simulink library "simulink"  (R2014a)
settings: Solver=ode45  SolverMode=SingleTasking  StartTime=0.0  StopTime=10.0  RelTol=1e-3
PostLoadFcn:
  | setsysloc_simulink(bdroot)
undefined symbols (not defined in the file or in its folder): DiscIntNeverNeededParam, getdatatypespecs, NumBits1, NumBits2, sfunxy, sigbuilder_block, slcm, SlDemoSign, Slope1, Slope2
libraries: simulink x40, sl_helperblocks x2, eml_lib x1
(part 3 of 5)

== system simulink/Model-Wide Utilities ==
  note: Linearization of Running Models
  note: Documentation
  note: Modeling Guides
  Block Support Table : Subsystem  mask(Block Support Table){}
      mask help: Simulink:masks:BlockSupportTable_MD
      settings: OpenFcn=showblockdatatypetable
      mask Display: disp('Block Support\nTable');
  DocBlock : Subsystem  mask(DocBlock){ECoderFlag=, DocumentType=Text}
      mask prompts: ECoderFlag "Simulink:masks:DocBlockEmbeddedCoderFlagLabel_MP"; DocumentType "Simulink:masks:DocBlockDocTypeLabel_MP"
      mask help: Simulink:masks:DocBlock_MD
      settings: DeleteFcn=docblock('close_document',gcb);  PreSaveFcn=docblock('save_document',gcb);  OpenFcn=docblock('edit_document',gcb);
      mask TypeOptions DocumentType: Simulink:masks:Text | Simulink:masks:RTF | Simulink:masks:HTML
      mask Display:
      | plot([.8 0 0 1 1 .8 .8 1],[1 1 0 0 .8 1 .8 .8]);
      | text(.5,.6,'DOC','horizontalalignment','center');
      | text(.95,.05,get_param(gcb,'DocumentType'),'verticalalignment','bottom','horizontalalignment','right');
  Model Info : Subsystem  LoadFcn=slcm LoadBlock;  InitFcn=slcm('UpdateAllCMBlocksInThisModelInit')  mask(CMBlock){InitialSaveTempField=, InitialBlockCM=None, BlockCM=none, Frame=on, SaveTempField=, DisplayStringWithTags=Model Info, MaskDisplayString=Model Info, HorizontalTextAlignment=Center, LeftAlignmentValue=0.5, SourceBlockDiagram=simulink, TagMaxNumber=20, CMTag1=, CMTag2=, CMTag3=, CMTag4=, CMTag5=, CMTag6=, CMTag7=, CMTag8=, CMTag9=, CMTag10=, CMTag11=, CMTag12=, CMTag13=, CMTag14=, CMTag15=, CMTag16=, CMTag17=, CMTag18=, CMTag19=, CMTag20=}
      mask prompts: InitialSaveTempField "Simulink:masks:InitialSaveTempField_MP"; InitialBlockCM "Simulink:masks:InitialBlockCM_MP"; BlockCM "Simulink:masks:BlockCM_MP"; Frame "Simulink:masks:Frame_MP"; SaveTempField "Simulink:masks:SaveTempField_MP"; DisplayStringWithTags "Simulink:masks:DisplayStringWithTags_MP"; MaskDisplayString "Simulink:masks:MaskDisplayString_MP"; HorizontalTextAlignment "Simulink:masks:HorizontalTextAlignment_MP"; LeftAlignmentValue "Simulink:masks:LeftAlignmentValue_MP"; SourceBlockDiagram "Simulink:masks:SourceBlockDiagram_MP"; TagMaxNumber "Simulink:masks:TagMaxNumber_MP"; CMTag1 "Simulink:masks:CMTag1_MP"; CMTag2 "Simulink:masks:CMTag2_MP"; CMTag3 "Simulink:masks:CMTag3_MP"; CMTag4 "Simulink:masks:CMTag4_MP"; CMTag5 "Simulink:masks:CMTag5_MP"; CMTag6 "Simulink:masks:CMTag6_MP"; CMTag7 "Simulink:masks:CMTag7_MP"; CMTag8 "Simulink:masks:CMTag8_MP"; CMTag9 "Simulink:masks:CMTag9_MP"; CMTag10 "Simulink:masks:CMTag10_MP"; CMTag11 "Simulink:masks:CMTag11_MP"; CMTag12 "Simulink:masks:CMTag12_MP"; CMTag13 "Simulink:masks:CMTag13_MP"; CMTag14 "Simulink:masks:CMTag14_MP"; CMTag15 "Simulink:masks:CMTag15_MP"; CMTag16 "Simulink:masks:CMTag16_MP"; CMTag17 "Simulink:masks:CMTag17_MP"; CMTag18 "Simulink:masks:CMTag18_MP"; CMTag19 "Simulink:masks:CMTag19_MP"; CMTag20 "Simulink:masks:CMTag20_MP"
      mask help: Simulink:masks:CMBlock_MD
      settings: CopyFcn=slcm CopyBlock;  DeleteFcn=slcm Cancel;  PostSaveFcn=slcm('UpdateAllCMBlocksInThisModel')  NameChangeFcn=slcm Rename;  OpenFcn=slcm
      mask Display: text(slResolve(LeftAlignmentValue, gcbh), 0.5, MaskDisplayString, 'HorizontalAlignment', HorizontalTextAlignment)
  Timed-Based Linearization : Subsystem  mask(Timed Linearization){LinearizationTime=1, SampleTime=0}
      mask prompts: LinearizationTime "Simulink:masks:LinearizationTime_MP"; SampleTime "Simulink:masks:SampleTimeofLinearizedModel_MP"
      mask help: Simulink:masks:TimedLinearization_MD
      mask init:
      | name_  = linsetup;
      mask Help: This block calls LINMOD or DLINMOD to create a linear model for the system when the simulation clock reaches the time specified by the LinearizationTime parameter.  No trimming is performed.  The linear model is stored in the base workspace as a structure, along with information about the operating point at which the snapshot was taken.  Multiple snapshots are appended to form an array of structures.
      mask Display: disp(['T=' mat2str(double(LinearizationTime))])
  Trigger-Based Linearization : Subsystem  TreatAsAtomicUnit=on  mask(Triggered Linearization){TriggerType=rising, SampleTime=0}
      mask prompts: TriggerType "Simulink:masks:TriggerType_MP"; SampleTime "Simulink:masks:SampleTimeofLinearizedModel_MP"
      mask help: Simulink:masks:TriggeredLinearization_MD
      mask init:
      | name_ = linsetup;
      | set_param([ gcb '/Trigger'],'TriggerType',TriggerType);
      mask Help: When triggered, this block calls LINMOD or DLINMOD to create a linear model for the system at the current operating point.  No trimming is performed.   The linear model is stored in the base workspace as a structure, along with information about the operating point at which the snapshot was taken.  Multiple snapshots are appended to form an array of structures.
      mask TypeOptions TriggerType: Simulink:masks:rising | Simulink:masks:falling | Simulink:masks:either | Simulink:masks:functionCall

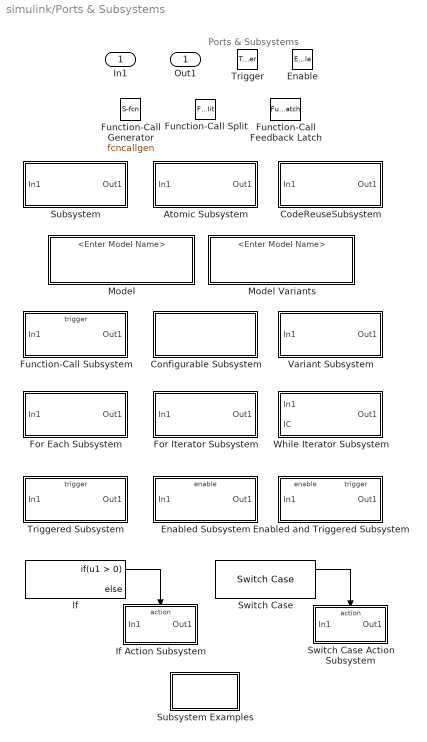
== system simulink/Ports & Subsystems ==
  note: Ports & Subsystems
  In1 : Inport
  Enable : EnablePort
  Trigger : TriggerPort  PortDimensions=1
  Atomic Subsystem : Subsystem  TreatAsAtomicUnit=on  mask(Atomic Subsystem){}
      mask help: Simulink:masks:IOPortSubsystem_MD
      settings: CopyFcn=set_param(gcbh,'LinkStatus','none'); set_param(gcbh,'Mask','off'); set_param(gcbh,'MaskType',''); set_param(gcbh,'MaskDescription',''); set_param(gcbh,'OpenFcn',''); set_param(gcbh,'CopyFcn','')  OpenFcn=open_system(gcbh,'force')
  CodeReuseSubsystem : Subsystem  TreatAsAtomicUnit=on  mask(Code Reuse Subsystem){}
      mask help: Simulink:masks:IOPortSubsystem_MD
      settings: CopyFcn=set_param(gcbh,'LinkStatus','none'); set_param(gcbh,'Mask','off'); set_param(gcbh,'MaskType',''); set_param(gcbh,'MaskDescription',''); set_param(gcbh,'OpenFcn',''); set_param(gcbh,'CopyFcn','')  OpenFcn=open_system(gcb,'force')  RTWFcnNameOpts=Use subsystem name  RTWFileNameOpts=Use function name
  Configurable Subsystem : Subsystem
      settings: TemplateBlock=master
  Enabled Subsystem : Subsystem  TreatAsAtomicUnit=on  mask(Enabled Subsystem){}
      mask help: Simulink:masks:EnabledSubsystem_MD
      settings: CopyFcn=set_param(gcbh,'LinkStatus','none'); set_param(gcbh,'Mask','off'); set_param(gcbh,'MaskType',''); set_param(gcbh,'MaskDescription',''); set_param(gcbh,'OpenFcn',''); set_param(gcbh,'CopyFcn','')  OpenFcn=open_system(gcbh,'force')
  Enabled and Triggered Subsystem : Subsystem  TreatAsAtomicUnit=on  mask(Enabled And Triggered Subsystem){}
      mask help: Simulink:masks:EnabledAndTriggeredSubsystem_MD
      settings: CopyFcn=set_param(gcbh,'LinkStatus','none'); set_param(gcbh,'Mask','off'); set_param(gcbh,'MaskType',''); set_param(gcbh,'MaskDescription',''); set_param(gcbh,'OpenFcn',''); set_param(gcbh,'CopyFcn','')  OpenFcn=open_system(gcbh,'force')
  For Each Subsystem : Subsystem  TreatAsAtomicUnit=on  mask(For Each Subsystem){}
      mask help: Simulink:masks:ForEachSubsystem_MD
      settings: CopyFcn=set_param(gcbh,'LinkStatus','none'); set_param(gcbh,'Mask','off'); set_param(gcbh,'MaskType',''); set_param(gcbh,'MaskDescription',''); set_param(gcbh,'OpenFcn',''); set_param(gcbh,'CopyFcn','')  OpenFcn=open_system(gcbh,'force')
  For Iterator Subsystem : Subsystem  TreatAsAtomicUnit=on  mask(For Iterator Subsystem){}
      mask help: Simulink:masks:ForIteratorSubsystem_MD
      settings: CopyFcn=set_param(gcbh,'LinkStatus','none'); set_param(gcbh,'Mask','off'); set_param(gcbh,'MaskType',''); set_param(gcbh,'MaskDescription',''); set_param(gcbh,'OpenFcn',''); set_param(gcbh,'CopyFcn','')  OpenFcn=open_system(gcbh,'force')
  Function-Call Feedback Latch : FunctionCallFeedbackLatch
  Function-Call Generator : S-Function  FunctionName=fcncallgen  Parameters=sample_time,numberOfIterations  EnableBusSupport=off  mask(Function-Call Generator){sample_time=1, numberOfIterations=1}
      mask prompts: sample_time "Simulink:masks:SampleTime_MP"; numberOfIterations "Simulink:masks:NumberOfIterations_MP"
      mask help: Simulink:masks:FunctionCallGenerator_MD
      mask init:
      | if ~isempty(numberOfIterations) & length(numberOfIterations) == 1 & (numberOfIterations > 1),
      | str=sprintf('iterate I = 1:%d',numberOfIterations);
      | else, str = 'f()';
      | end;
      mask Help: This block executes a function-call subsystem at the rate specified by the sample time and a specified number of times.
      mask Display: disp(str)
  Function-Call Split : FunctionCallSplit
      settings: CopyFcn=set_param(gcbh,'ShowName','off','CopyFcn','')
  Function-Call Subsystem : Subsystem  TreatAsAtomicUnit=on  mask(Function-Call Subsystem){}
      mask help: Simulink:masks:FunctionCallSubsystem_MD
      settings: CopyFcn=set_param(gcbh,'LinkStatus','none'); set_param(gcbh,'Mask','off'); set_param(gcbh,'MaskType',''); set_param(gcbh,'MaskDescription',''); set_param(gcbh,'OpenFcn',''); set_param(gcbh,'CopyFcn','')  OpenFcn=open_system(gcbh,'force')
  If : If
  If Action Subsystem : Subsystem  TreatAsAtomicUnit=on  mask(If Action Subsystem){}
      mask help: Simulink:masks:ActionSubsystem_MD
      settings: CopyFcn=set_param(gcbh,'LinkStatus','none'); set_param(gcbh,'Mask','off'); set_param(gcbh,'MaskType',''); set_param(gcbh,'MaskDescription',''); set_param(gcbh,'OpenFcn',''); set_param(gcbh,'CopyFcn','')  OpenFcn=open_system(gcbh,'force')
  Model : ModelReference  ModelNameDialog=<Enter Model Name>  SimulationMode=Normal  DefaultDataLogging=on
  Model Variants : ModelReference  ModelNameDialog=<Enter Model Name>  SimulationMode=Normal  Variant=on  DefaultDataLogging=on
      settings: AttributesFormatString=%<ActiveVariant>
  Subsystem : Subsystem  mask(Virtual Subsystem){}
      mask help: Simulink:masks:IOPortSubsystem_MD
      settings: CopyFcn=set_param(gcbh,'LinkStatus','none'); set_param(gcbh,'Mask','off'); set_param(gcbh,'MaskType',''); set_param(gcbh,'MaskDescription',''); set_param(gcbh,'OpenFcn',''); set_param(gcbh,'CopyFcn','')  OpenFcn=open_system(gcbh,'force')
  Subsystem Examples : Subsystem  mask(Subsystem Examples){}
      mask help: Simulink:masks:SubsystemExamples_MD
      settings: OpenFcn=open_system('sl_subsys_semantics','force')
      mask Display: disp('Subsystem\nExamples')
  Switch Case : SwitchCase
  Switch Case Action Subsystem : Subsystem  TreatAsAtomicUnit=on  mask(Switch Case Action Subsystem){}
      mask help: Simulink:masks:ActionSubsystem_MD
      settings: CopyFcn=set_param(gcbh,'LinkStatus','none'); set_param(gcbh,'Mask','off'); set_param(gcbh,'MaskType',''); set_param(gcbh,'MaskDescription',''); set_param(gcbh,'OpenFcn',''); set_param(gcbh,'CopyFcn','')  OpenFcn=open_system(gcbh,'force')
  Triggered Subsystem : Subsystem  TreatAsAtomicUnit=on  mask(Triggered Subsystem){}
      mask help: Simulink:masks:TriggeredSubsystem_MD
      settings: CopyFcn=set_param(gcbh,'LinkStatus','none'); set_param(gcbh,'Mask','off'); set_param(gcbh,'MaskType',''); set_param(gcbh,'MaskDescription',''); set_param(gcbh,'OpenFcn',''); set_param(gcbh,'CopyFcn','')  OpenFcn=open_system(gcbh,'force')
  Variant Subsystem : Subsystem  Variant=on  mask(Variant Subsystem){}
      mask help: Simulink:masks:VariantSubsystem_MD
      settings: CopyFcn=set_param(gcbh,'LinkStatus','none'); set_param(gcbh,'Mask','off'); set_param(gcbh,'MaskType',''); set_param(gcbh,'MaskDescription',''); set_param(gcbh,'OpenFcn',''); set_param(gcbh,'CopyFcn','')
  While Iterator Subsystem : Subsystem  TreatAsAtomicUnit=on  mask(While Iterator Subsystem){}
      mask help: Simulink:masks:WhileIteratorSubsystem_MD
      settings: CopyFcn=set_param(gcbh,'LinkStatus','none'); set_param(gcbh,'Mask','off'); set_param(gcbh,'MaskType',''); set_param(gcbh,'MaskDescription',''); set_param(gcbh,'OpenFcn',''); set_param(gcbh,'CopyFcn','')  OpenFcn=open_system(gcbh,'force')
  Out1 : Outport
  wires:
  If/1 -> If Action Subsystem/Action
  Switch Case/1 -> Switch Case Action Subsystem/Action

== system simulink/Signal Attributes ==
  note: Signal Attribute Manipulation
  note: Signal Attribute Detection
  Bus to Vector : BusToVector
  Data Type Conversion Inherited : Subsystem  mask(Conversion Inherited){ConvertRealWorld=Real World Value, RndMeth=Floor, DoSatur=off}
      mask prompts: ConvertRealWorld "Simulink:masks:InputAndOutputToHaveEqual_MP"; RndMeth "Simulink:masks:IntegerRoundingMode_MP"; DoSatur "Simulink:masks:SaturateToMaxOrMinWhenOverflowsOccur_MP"
      mask help: Simulink:masks:ConversionInherited_MD
      mask init:
      | rndMethCell = {'Ceiling','Convergent','Floor','Nearest','Round','Simplest','Zero'};
      | onOffCell = {'off','on'};
      | RWVvsSICell = { 'Real World Value','Stored Integer'};
      | set_param([gcb,'/Conversion'],'RndMeth',rndMethCell{RndMeth},...
      |                                 'DoSatur',onOffCell{DoSatur+1},...
      |                                 'ConvertRealWorld',RWVvsSICell{ConvertRealWorld});
      mask TypeOptions ConvertRealWorld: Simulink:masks:RealWorldValue | Simulink:masks:StoredInteger
      mask TypeOptions RndMeth: Simulink:masks:Ceiling | Simulink:masks:Convergent | Simulink:masks:Floor | Simulink:masks:Nearest | Simulink:masks:Round | Simulink:masks:Simplest | Simulink:masks:Zero
      mask Display:
      | port_label('Input',2,'u');
      | port_label('Output',1,'y');
      | disp('Convert')
  Data Type Duplicate : DataTypeDuplicate
  Data Type Propagation : S-Function  FunctionName=sfix_dtprop  Parameters=14,PropDataTypeMode,(getdatatypespecs(PropDataType,PropScaling,DblOver,0, 0, PropDataTypeMode, PropScalingMode)),IfRefDouble,IfRefSingle,IsSigned,NumBitsBase,NumBitsMult,NumBitsAdd,(sort(reshape(round(NumBitsAllowFinal), prod(size(NumBitsAllowFinal)),1))),PropScalingMode,ValuesUsedBestPrec,SlopeBase,SlopeMult,SlopeAdd,BiasBase,BiasMult,BiasAdd,DblOver  EnableBusSupport=off  mask(Data Type Propagation){PropDataTypeMode=Inherit via propagation rule, PropDataType=fixdt(1, 16), IfRefDouble=double, IfRefSingle=single, IsSigned=IsSigned1 or IsSigned2, NumBitsBase=max([NumBits1 NumBits2]), NumBitsMult=1, NumBitsAdd=0, NumBitsAllowFinal=1:128, PropScalingMode=Inherit via propagation rule, PropScaling=2^-10, ValuesUsedBestPrec=[5 -7], SlopeBase=min([Slope1 Slope2]), SlopeMult=1, SlopeAdd=0, BiasBase=Bias1, BiasMult=1, BiasAdd=0}
      mask prompts: PropDataTypeMode "Simulink:masks:x1PropagatedDataType_MP"; PropDataType "Simulink:masks:x11PropagatedDataTypeegFixdt116Fixdtsingle_MP"; IfRefDouble "Simulink:masks:x11IfAnyReferenceInputIsDoubleOutputIs_MP"; IfRefSingle "Simulink:masks:x12IfAnyReferenceInputIsSingleOutputIs_MP"; IsSigned "Simulink:masks:x13IsSigned_MP"; NumBitsBase "Simulink:masks:x141NumberofBitsBase_MP"; NumBitsMult "Simulink:masks:x142NumberofBitsMultiplicativeAdjustment_MP"; NumBitsAdd "Simulink:masks:x143NumberofBitsAdditiveAdjustment_MP"; NumBitsAllowFinal "Simulink:masks:x144NumberofBitsAllowableFinalValues_MP"; PropScalingMode "Simulink:masks:x2PropagatedScaling_MP"; PropScaling "Simulink:masks:x21PropagatedScalingSlopeEg29OrSlopeBiasEg1253_MP"; ValuesUsedBestPrec "Simulink:masks:x21ValuesUsedToDetermineBestPrecisionScaling_MP"; SlopeBase "Simulink:masks:x211SlopeBase_MP"; SlopeMult "Simulink:masks:x212SlopeMultiplicativeAdjustment_MP"; SlopeAdd "Simulink:masks:x213SlopeAdditiveAdjustment_MP"; BiasBase "Simulink:masks:x221BiasBase_MP"; BiasMult "Simulink:masks:x222BiasMultiplicativeAdjustment_MP"; BiasAdd "Simulink:masks:x223BiasAdditiveAdjustment_MP"
      mask help: Simulink:masks:DataTypePropagation_MD
      mask init:
      | DblOver = 0;
      mask TypeOptions PropDataTypeMode: Simulink:masks:SpecifyViaDialog | Simulink:masks:InheritViaPropagationRule
      mask Callback PropDataTypeMode: fixptdialog(gcbh)
      mask Callback PropDataType: fixptdialog(gcbh)
      mask TypeOptions IfRefDouble: Simulink:masks:double | Simulink:masks:single
      mask TypeOptions IfRefSingle: Simulink:masks:double | Simulink:masks:single
      mask TypeOptions IsSigned: Simulink:masks:IsSigned1 | Simulink:masks:IsSigned2 | Simulink:masks:IsSigned1OrIsSigned2 | Simulink:masks:TRUE | Simulink:masks:FALSE
      mask TypeOptions NumBitsBase: NumBits1 | NumBits2 | max([NumBits1 NumBits2]) | min([NumBits1 NumBits2]) | NumBits1+NumBits2
      mask TypeOptions PropScalingMode: Simulink:masks:SpecifyViaDialog | Simulink:masks:InheritViaPropagationRule | Simulink:masks:ObtainViaBestPrecision
      mask Callback PropScalingMode: fixptdialog(gcbh)
      mask TypeOptions SlopeBase: Slope1 | Slope2 | max([Slope1 Slope2]) | min([Slope1 Slope2]) | Slope1*Slope2 | Slope1/Slope2 | PosRange1 | PosRange2 | max([PosRange1 PosRange2]) | min([PosRange1 PosRange2]) | PosRange1*PosRange2 | PosRange1/PosRange2
      mask TypeOptions BiasBase: Bias1 | Bias2 | max([Bias1 Bias2]) | min([Bias1 Bias2]) | Bias1*Bias2 | Bias1/Bias2 | Bias1+Bias2 | Bias1-Bias2
      mask Display:
      | port_label('Input',1,'Ref1');
      | port_label('Input',2,'Ref2');
      | port_label('Input',3,'Prop');
  Data Type Propagation Examples : Subsystem  mask(Data Type Propagation Examples){}
      mask help: Simulink:masks:DataTypePropagationExamples_MD
      settings: OpenFcn=open_system('fixpt_dtprop','force')
      mask Display: disp('Data Type\nPropagation\nExamples')
  Data Type Scaling Strip : Subsystem  mask(Scaling Strip){}
      mask help: Simulink:masks:ScalingStrip_MD
      mask Display: fprintf('Scaling\nStrip')
  Data Type Conversion : DataTypeConversion
  IC : InitialCondition
  Probe : Probe  ProbeSignalDimensions=on  ProbeFramedSignal=on
  Rate Transition : RateTransition
  Signal Conversion : SignalConversion
  Signal Specification : SignalSpecification
  Weighted Sample Time : SampleTimeMath  TsampMathOp=Ts Only
  Width : Width

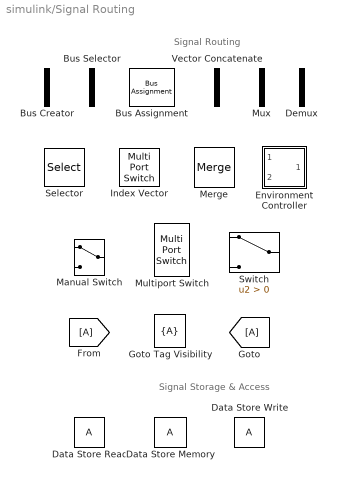
== system simulink/Signal Routing ==
  note: Signal Routing
  note: Signal Storage & Access
  Bus Assignment : BusAssignment
  Bus Creator : BusCreator  Inputs=2
      settings: CopyFcn=set_param(gcbh,'ShowName','off','CopyFcn','')
  Bus Selector : BusSelector  OutputSignals=signal1,signal2
      settings: CopyFcn=set_param(gcbh,'ShowName','off','CopyFcn','')
  Data Store Memory : DataStoreMemory  ReadBeforeWriteMsg=warning  WriteAfterWriteMsg=warning  WriteAfterReadMsg=warning
  Data Store Read : DataStoreRead
  Data Store Write : DataStoreWrite
  Demux : Demux  Outputs=2
      settings: CopyFcn=set_param(gcbh,'ShowName','off','CopyFcn','')
  Environment Controller : Subsystem  mask(Environment Controller){}
      mask help: Simulink:masks:EnvironmentController_MD
      mask init:
      | switch_mode = rtwenvironmentmode(bdroot(gcbh)) || ...
      |     (exist('sldvisactive','file')~=0 && sldvisactive(bdroot(gcbh)));
  Goto Tag Visibility : GotoTagVisibility
  Index Vector : MultiPortSwitch  DataPortOrder=Zero-based contiguous  Inputs=1  zeroidx=on
  Manual Switch : ManualSwitch
  Merge : Merge
  Multiport Switch : MultiPortSwitch
  Mux : Mux  Inputs=2
      settings: CopyFcn=set_param(gcbh,'ShowName','off','CopyFcn','')
  Selector : Selector  InputPortWidth=3  Indices=[1 3]
  Switch : Switch  Criteria=u2 > Threshold
  Vector Concatenate : Concatenate

== system simulink/Sinks ==
  note: Model & Subsystem Outputs
  note: Simulation Control
  note: Data Viewers
  Display : Display
  Floating Scope : Scope
      settings: Floating=on
  Scope : Scope
  Stop Simulation : Stop
  Terminator : Terminator
  To File : ToFile  SaveFormat=Timeseries
  To Workspace : ToWorkspace  VariableName=simout  SaveFormat=Timeseries  SampleTime=-1
  XY Graph : Subsystem  LoadFcn=sfunxy([],[],[],'LoadBlock')  StartFcn=sfunxy([],[],[],'Start')  StopFcn=sfunxy([],[],[],'Stop')  TreatAsAtomicUnit=on  SimViewingDevice=on  mask(XY scope.){xmin=-1, xmax=1, ymin=-1, ymax=1, st=-1}
      mask prompts: xmin "Simulink:masks:xmin_MP"; xmax "Simulink:masks:xmax_MP"; ymin "Simulink:masks:ymin_MP"; ymax "Simulink:masks:ymax_MP"; st "Simulink:masks:SampleTime_MP"
      mask help: Simulink:masks:XYScope_MD
      settings: CopyFcn=sfunxy([],[],[],'CopyBlock')  DeleteFcn=sfunxy([],[],[],'DeleteBlock')  NameChangeFcn=sfunxy([],[],[],'NameChange')
      mask Help: This block can be used to explore limit cycles. Look at the m-file sfunxy.m to see how it works.
      mask Display: plot([.05 .95 .95 .05 .05],[.45 .45 .95 .95 .45], 0.5+cos(0:0.1:2*pi)*0.3,0.7+sin(0:0.1:2*pi)*0.2)
  Out1 : Outport

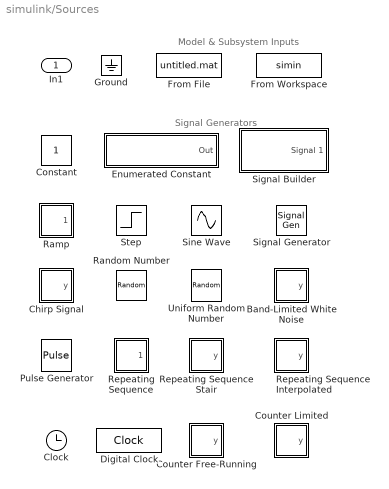
== system simulink/Sources ==
  note: Model & Subsystem Inputs
  note: Signal Generators
  In1 : Inport
  Band-Limited White Noise : Subsystem  mask(Band-Limited White Noise.){Cov=[0.1], Ts=0.1, seed=[23341], VectorParams1D=on}
      mask prompts: Cov "Simulink:masks:NoisePower_MP"; Ts "Simulink:masks:SampleTime_MP"; seed "Simulink:masks:Seed_MP"; VectorParams1D "Simulink:masks:InterpretVectorParametersAs1D_MP"
      mask help: Simulink:masks:BandLimitedWhiteNoise_MD
      mask init:
      | if any(Cov < 0),
      | 	error('The ''Noise power'' must be positive. '),
      | end;
      | 
      | r = [-0.4326
      |    -1.6656
      |     0.1253
      |     0.2877
      |    -1.1465
      |     1.1909
      |     1.1892
      |    -0.0376
      |     0.3273
      |     0.1746
      |    -0.1867
      |     0.7258]';
      | 
      | r2 = [r(1),r;r,r(12)]; 
      | t =[1:13;1:13]; 
      | 
      | if any(Ts==-1), 
      | 	error('Sample time (-1) is set to be back-inherited from the block(s) it drives. You should explicitly specify the sample time of the source block. '), 
      | end;
      | set_param([gcb '/White Noise'],'VectorParams1D',VectorParams1D);
      mask Help: Implemented using white noise into Zero-Order Hold block. The seed and power can be vectors of the same length to produce a vector of white noise sources. For faster simulation, set sample time to the highest value possible but in accordance with the fastest dynamics of system.
      mask Display: plot(t(:),r2(:))
  Chirp Signal : Subsystem  mask(chirp){f1=0.1, T=100, f2=1, VectorParams1D=on}
      mask prompts: f1 "Simulink:masks:InitialFrequencyHz_MP"; T "Simulink:masks:TargetTimesecs_MP"; f2 "Simulink:masks:FrequencyAtTargetTimeHz_MP"; VectorParams1D "Simulink:masks:InterpretVectorParametersAs1D_MP"
      mask help: Simulink:masks:chirp_MD
      mask init:
      | blkName = gcb;
      | t=[0:.1:5];
      | set_param([blkName '/targetTime'], 'VectorParams1D', VectorParams1D);
      | set_param([blkName '/initialFreq'], 'VectorParams1D', VectorParams1D);
      | set_param([blkName '/deltaFreq'], 'VectorParams1D', VectorParams1D);
      mask Help: The chirp signal has linearly increasing frequency with time.  This block can be used for spectral analysis of nonlinear systems.
      mask Display: plot(t,sin(t.*t))
  Clock : Clock
  Constant : Constant
  Counter Free-Running : Subsystem  mask(Counter Free-Running){NumBits=16, tsamp=-1}
      mask prompts: NumBits "Simulink:masks:NumberOfBits_MP"; tsamp "Simulink:masks:SampleTime_MP"
      mask help: Simulink:masks:CounterFreeRunning_MD
      mask Display: plot( 0.05+0.9/8*[0 1 1 2 2 3 3 4 4 5 5 6 6 7 7 8 8], 0.3+0.65/3*[0 0 1 1 2 2 3 3 0 0 1 1 2 2 3 3 0] )
  Counter Limited : Subsystem  mask(Counter Limited){uplimit=7, tsamp=-1}
      mask prompts: uplimit "Simulink:masks:UpperLimit_MP"; tsamp "Simulink:masks:SampleTime_MP"
      mask help: Simulink:masks:CounterLimited_MD
      mask init:
      | nbits = sl('counter_init', uplimit, gcbh);
      mask Display:
      | plot( 0.15+0.8/8*[0 1 1 2 2 3 3 4 4 5 5 6 6 7 7 8 8], 0.3+0.65/3*[0 0 1 1 2 2 3 3 0 0 1 1 2 2 3 3 0] )
      | text(0.05,0.85,'lim')
  Digital Clock : DigitalClock
  Enumerated Constant : Subsystem  DialogController=Simulink.DDGSource  mask(Enumerated Constant){OutDataTypeStr=Enum: SlDemoSign, Value=SlDemoSign.Positive, SampleTime=inf}
      mask prompts: OutDataTypeStr "Simulink:masks:OutputDataType_MP"; Value "Simulink:masks:Value_MP"; SampleTime "Simulink:masks:SampleTime_MP"
      mask init:
      | % NOTE:
      | % Value is not evaluated to avoid caching an instance
      | % of the MCOS class by the mask infrastructure.
      | 
      | % Get string to use for display purposes
      | enumConstDispStr = Value;
      | if isempty(enumConstDispStr)
      |   enumConstDispStr = '???';
      | end
      | 
      | % Check data type & value
      | enumconst_cb('MaskInit', OutDataTypeStr, slResolve(Value, gcb));
      | 
      | % Set mask parameter values directly on underlying block
      | % and clear mask workspace variables to prevent underlying
      | % blocks from resolving to unevaluated mask variables.
      | set_param([gcb, '/Constant'], ...
      |     'OutDataTypeStr', OutDataTypeStr, ...
      |     'SampleTime',     SampleTime, ...
      |     'Value',          Value);
      | clear OutDataTypeStr SampleTime Value;
      mask Display: disp(enumConstDispStr)
  From Workspace : FromWorkspace  VariableName=simin  SampleTime=0
  From File : FromFile  SampleTime=0
  Ground : Ground
  Pulse Generator : DiscretePulseGenerator  PulseType=Time based  Period=10  PulseWidth=5
  Ramp : Subsystem  mask(Ramp){slope=1, start=0, X0=0, VectorParams1D=on}
      mask prompts: slope "Simulink:masks:Slope_MP"; start "Simulink:masks:StartTime_MP"; X0 "Simulink:masks:InitialOutput_MP"; VectorParams1D "Simulink:masks:InterpretVectorParametersAs1D_MP"
      mask help: Simulink:masks:Ramp_MD
      mask init:
      | blkName = gcb;
      | set_param([blkName '/Constant'], 'VectorParams1D',VectorParams1D);
      | set_param([blkName '/Constant1'], 'VectorParams1D',VectorParams1D);
      | set_param([blkName '/Step'], 'VectorParams1D',VectorParams1D);
      mask Display: plot([2,4,8],[0,0,4])
  Random Number : RandomNumber  SampleTime=0.1
  Repeating Sequence : Subsystem  mask(Repeating table){rep_seq_t=[0 2], rep_seq_y=[0 2]}
      mask prompts: rep_seq_t "Simulink:masks:TimeValues_MP"; rep_seq_y "Simulink:masks:OutputValues_MP"
      mask help: Simulink:masks:RepeatingTable_MD
      mask init:
      | X = [];
      | Y = [];
      | if (length(rep_seq_t) ~= length(rep_seq_y)),
      |   error('Length of time vector and output vector must be the same.')
      | end
      | dbl_rep_seq_t = double(rep_seq_t);
      | dbl_rep_seq_y = double(rep_seq_y);
      | period = max(dbl_rep_seq_t) - min(dbl_rep_seq_t);
      | period = slResolve(sprintf('%0.5g',period), gcbh);
      | [X, Y] = genRepeatingSequenceBlockIconData(dbl_rep_seq_t, dbl_rep_seq_y);
      mask Help: Repeats cycle given in table. Time values should be monotonically increasing.
      mask Display: plot(X, Y )
  Repeating Sequence Interpolated : Subsystem  mask(Repeating Sequence Interpolated){OutValues=[3 1 4 2 1].', TimeValues=[0 0.1 0.5 0.6 1].', LookUpMeth=Interpolation-Use End Values, tsamp=0.01, OutMin=[], OutMax=[], OutDataTypeStr=double, OutputDataTypeScalingMode=double, OutDataType=fixdt(0,8), OutScaling=2^-10, LockScale=off}
      mask prompts: OutValues "Simulink:masks:VectorOfOutputValues_MP"; TimeValues "Simulink:masks:VectorOfTimeValues_MP"; LookUpMeth "Simulink:masks:LookupMethod_MP"; tsamp "Simulink:masks:SampleTime_MP"; OutMin "Simulink:masks:OutputMinimum_MP"; OutMax "Simulink:masks:OutputMaximum_MP"; OutDataTypeStr "Simulink:masks:OutputDataType_MP"; OutputDataTypeScalingMode "Simulink:masks:OutputDataTypeMode_MP"; OutDataType "Simulink:masks:OutputDataTypeegFixdt116Fixdtsingle_MP"; OutScaling "Simulink:masks:OutputScalingSlopeEg29OrSlopeBias_MP"; LockScale "Simulink:masks:LockOutputDataTypeAgainstFxpTools_MP"
      mask help: Simulink:masks:RepeatingSequenceInterpolated_MD
      mask init:
      | X = [];
      | Y = [];
      | xx = double(TimeValues);
      | yy = double(OutValues);
      | if min(xx) < 0
      |   error('Negative Time Values are not supported.');
      |   xx = [];
      | elseif min(xx) > 0
      |   xx(2:(end+1)) = xx;
      |   xx(1) = 0;
      |   yy(2:(end+1)) = yy;
      | end
      | if tsamp == -1
      |   tsamp = min(diff(xx));
      | end
      | nn = floor(max(xx)/double(tsamp));
      | 
      | [X, Y] = genRepeatingSequenceInterpolatedBlockIconData(xx, yy, LookUpMeth);
      | 
      | LookupMethod = get_param(gcb, 'LookupMeth');
      | 
      | switch LookupMethod
      |     case 'Interpolation-Use End Values'
      |         set_param([gcb, '/Lookup'], 'InterpMethod', 'Linear');
      |         set_param([gcb, '/Lookup'], 'ExtrapMethod', 'Clip');
      |     case 'Use Input Nearest'
      |         set_param([gcb, '/Lookup'], 'InterpMethod', 'Nearest');
      |     case 'Use Input Below'
      |         set_param([gcb, '/Lookup'], 'InterpMethod', 'Flat');    
      |     case 'Use Input Above'
      |         set_param([gcb, '/Lookup'], 'InterpMethod', 'Above');  
      | end
      mask TypeOptions LookUpMeth: Simulink:masks:InterpolationUseEndValues | Simulink:masks:UseInputNearest | Simulink:masks:UseInputBelow | Simulink:masks:UseInputAbove
      mask Callback OutDataTypeStr: fixptdialog(gcbh)
      mask TypeOptions OutputDataTypeScalingMode: double | single | int8 | uint8 | int16 | uint16 | int32 | uint32 | Specify via dialog | Inherit via back propagation
      mask Callback OutputDataTypeScalingMode: fixptdialog(gcbh)
      mask Callback OutDataType: fixptdialog(gcbh)
      mask Display: plot(X,Y)
  Repeating Sequence Stair : Subsystem  mask(Repeating Sequence Stair){OutValues=[3 1 4 2 1].', tsamp=-1, OutMin=[], OutMax=[], OutDataTypeStr=double, OutputDataTypeScalingMode=double, OutDataType=fixdt(0,8), ConRadixGroup=Best Precision: Vector-wise, OutScaling=2^-12, LockScale=off}
      mask prompts: OutValues "Simulink:masks:VectorOfOutputValues_MP"; tsamp "Simulink:masks:SampleTime_MP"; OutMin "Simulink:masks:OutputMinimum_MP"; OutMax "Simulink:masks:OutputMaximum_MP"; OutDataTypeStr "Simulink:masks:OutputDataType_MP"; OutputDataTypeScalingMode "Simulink:masks:OutputDataTypeMode_MP"; OutDataType "Simulink:masks:OutputDataTypeegFixdt116Fixdtsingle_MP"; ConRadixGroup "Simulink:masks:OutputScalingMode_MP"; OutScaling "Simulink:masks:OutputScalingSlopeEg29OrSlopeBias_MP"; LockScale "Simulink:masks:LockOutputDataTypeAgainstFxpTools_MP"
      mask help: Simulink:masks:RepeatingSequenceStair_MD
      mask init:
      | blk = gcb;
      | nn = length(OutValues)-1;
      | dim = size(OutValues);
      | if length(dim) > 2 || min(dim) ~= 1
      |   [X, Y] =  generateQuestionMarkIconData;
      |   error('Parameter ''output values'' must be a vector or a scalar');
      | else
      |   [X, Y] = genRepeatingSequenceStairBlockIconData(OutValues);
      | end
      | set_param([blk, '/', 'Output'], 'MarkFixedInMinorTimeSteps', 'on');
      mask Callback OutDataTypeStr: fixptdialog(gcbh)
      mask TypeOptions OutputDataTypeScalingMode: double | single | int8 | uint8 | int16 | uint16 | int32 | uint32 | Specify via dialog | Inherit via back propagation
      mask Callback OutputDataTypeScalingMode: fixptdialog(gcbh)
      mask Callback OutDataType: fixptdialog(gcbh)
      mask TypeOptions ConRadixGroup: Use specified scaling | Best Precision: Vector-wise
      mask Callback ConRadixGroup: fixptdialog(gcbh)
      mask Display: plot(X,Y)
  Signal Generator : SignalGenerator  Units=rad/sec
  Signal Builder : Subsystem  Tag=STV Subsys  LoadFcn=sigbuilder_block('load');  StartFcn=sigbuilder_block('start');  StopFcn=sigbuilder_block('stop');  ClipboardFcn=sigbuilder_block('clipboard');  mask(Sigbuilder block){}
      mask help: Simulink:masks:SigbuilderBlock_MD
      mask init:
      | if ~strcmp(get_param(bdroot(gcbh),'SimulationStatus'),'stopped') tuvar = sigbuilder_block('maskInit'); end
      settings: CopyFcn=sigbuilder_block('copy');  DeleteFcn=sigbuilder_block('delete');  ModelCloseFcn=sigbuilder_block('modelClose');  PreSaveFcn=sigbuilder_block('preSave');  PauseFcn=sigbuilder_block('pause');  ContinueFcn=sigbuilder_block('continue');  NameChangeFcn=sigbuilder_block('namechange');  OpenFcn=sigbuilder_block('open',[437.6 199.2 550.4 400 ]);  CloseFcn=sigbuilder_block('close');
      mask Display: plot(0, 0, 100, 100,[2, 2, 32, 32, 2], [68, 8, 8, 68, 68],[32, 2], [38, 38], [32, 19, 2],[53, 60, 44], [32, 17, 17, 2],[16, 16, 31, 31]);txt = getActiveGroup(gcbh);text(2, 100, txt,'verticalAlignment', 'top');
  Sine Wave : Sin  SampleTime=0
  Step : Step  SampleTime=0
  Uniform Random Number : UniformRandomNumber  SampleTime=0.1

== system simulink/User-Defined Functions ==
  note: User-defined Functions
  Fcn : Fcn  Expr=sin(u(1)*exp(2.3*(-u(2))))
  Interpreted MATLAB Function : MATLABFcn
  Level-2 MATLAB S-Function : M-S-Function
  MATLAB Function : eml_lib/MATLAB Function
  MATLAB System : MATLABSystem
  S-Function : S-Function  EnableBusSupport=off
  S-Function Builder : S-Function  EnableBusSupport=off  mask(S-Function Builder){}
      mask help: Simulink:masks:SFunctionBuilder_MD
      mask init:
      | val = [[.9  0.75 0.75 1 1 .9 .9 1]',[1 1 0.75 0.75 .9 .9 1 .9]'];
      | sys = get_param(gcbh,'FunctionName');
      settings: CopyFcn=set_param(gcbh,'LinkStatus','none')  OpenFcn=sfunctionwizard(gcbh)
      mask Display:
      | plot(val(:,1),val(:,2))
      | disp(sys)
  S-Function Examples : Subsystem  mask(S-Function Examples){}
      mask help: Simulink:masks:SFunctionExamples_MD
      settings: OpenFcn=open_system('sfundemos','force')
      mask Display: disp('S-Function\nExamples')

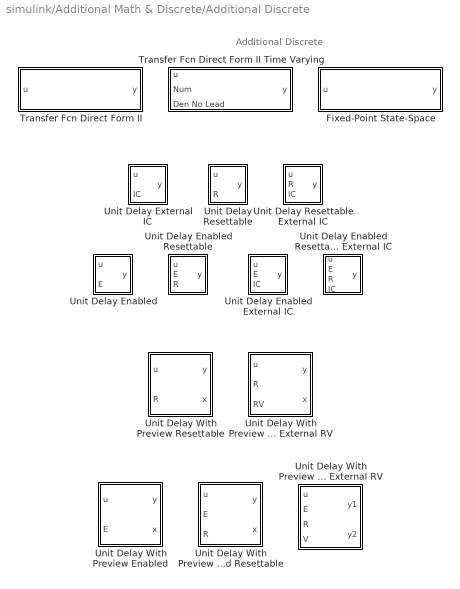
== system simulink/Additional Math & Discrete/Additional Discrete ==
  note: Additional Discrete
  Fixed-Point State-Space : Subsystem  mask(Fixed-Point State-Space){A=[2.6020 -2.2793 0.6708; 1 0 0; 0 1 0], B=[ 1; 0; 0], C=[0.0184    0.0024    0.0055], D=[0.0033], X0=0.0, InternalDataType=fixdt('double'), StateEqScaling=2^0, OutputEqScaling=2^0, LockScale=off, RndMeth=Floor, DoSatur=off}
      mask prompts: A "Simulink:masks:StateMatrixA_MP"; B "Simulink:masks:InputMatrixB_MP"; C "Simulink:masks:OutputMatrixC_MP"; D "Simulink:masks:DirectFeedthroughMatrixD_MP"; X0 "Simulink:masks:InitialConditionForState_MP"; InternalDataType "Simulink:masks:DataTypeForInternalCalculations_MP"; StateEqScaling "Simulink:masks:ScalingForStateEquationAXBU_MP"; OutputEqScaling "Simulink:masks:ScalingForOutputEquationCXDU_MP"; LockScale "Simulink:masks:LockOutputDataTypeAgainstFxpTools_MP"; RndMeth "Simulink:masks:IntegerRoundingMode_MP"; DoSatur "Simulink:masks:SaturateToMaxOrMinWhenOverflowsOccur_MP"
      mask help: Simulink:masks:FixedPointStateSpace_MD
      mask init:
      | blkH = gcbh;
      | blkName = getfullname(blkH);
      | 
      | vRndMeth = get_param(blkH,'RndMeth');
      | vDoSatur = get_param(blkH,'DoSatur');
      | blks = {'State Matrix A','Input Matrix B','Output Matrix C','Direct Link Matrix D','Sum Output Equation','Sum State Equation','Downcast Next State X','Downcast Output Y'};
      | for i = 1:length(blks)
      |   set_param([blkName,'/',blks{i}],'RndMeth',vRndMeth, ...
      | 	  'DoSatur',vDoSatur);
      | end
      mask TypeOptions RndMeth: Simulink:masks:Ceiling | Simulink:masks:Convergent | Simulink:masks:Floor | Simulink:masks:Nearest | Simulink:masks:Round | Simulink:masks:Simplest | Simulink:masks:Zero
      mask Display:
      | text(0.5, 0.5, 'y(n)=Cx(n)+Du(n)', 'horizontalAlignment', 'center', 'verticalAlignment', 'bottom');
      | text(0.5, 0.5, 'x(n+1)=Ax(n)+Bu(n)', 'horizontalAlignment', 'center', 'verticalAlignment', 'top');
  Transfer Fcn Direct Form II : Subsystem  mask(Transfer Fcn Direct Form II){NumCoefVec=[0.2 0.3 0.2], DenCoefVec=[-0.9    0.6], vinit=0.0, RndMeth=Floor, DoSatur=off}
      mask prompts: NumCoefVec "Simulink:masks:NumeratorCoefficients_MP"; DenCoefVec "Simulink:masks:DenominatorCoefficientsExcludingLead_MP"; vinit "Simulink:masks:InitialCondition_MP"; RndMeth "Simulink:masks:IntegerRoundingMode_MP"; DoSatur "Simulink:masks:SaturateToMaxOrMinWhenOverflowsOccur_MP"
      mask help: Simulink:masks:TransferFcnDirectFormII_MD
      mask init:
      | blkH = gcbh;
      | blkName = getfullname(blkH);
      | 
      | vRndMeth = get_param(blkH,'RndMeth');
      | vDoSatur = get_param(blkH,'DoSatur');
      | DCGain = polyval(NumCoefVec,1)./polyval([1 DenCoefVec],1);
      | maxGain = max( 1, max(max(abs(DCGain))) );
      | maxGain = max( maxGain, abs(NumCoefVec(1)) );
      | OutputSlopeMult = 2^ceil(log2(maxGain));
      | DCGain = (1)./polyval([1 DenCoefVec],1);
      | maxGain = max( 1, max(max(abs(DCGain))) );
      | OutputSlopeMult2 = 2^ceil(log2(maxGain));
      | set_param([blkName,'/NumCoef'],'RndMeth',vRndMeth, ...
      | 	'DoSatur',vDoSatur);
      | set_param([blkName,'/DenCoef'],'RndMeth',vRndMeth, ...
      | 	'DoSatur',vDoSatur);
      | set_param([blkName,'/Downcast'],'RndMeth',vRndMeth, ...
      | 	'DoSatur',vDoSatur);
      | set_param([blkName,'/Downcast1'],'RndMeth',vRndMeth, ...
      | 	'DoSatur',vDoSatur);
      | set_param([blkName,'/Sum'],'RndMeth',vRndMeth, ...
      | 	'DoSatur',vDoSatur);
      mask TypeOptions RndMeth: Simulink:masks:Ceiling | Simulink:masks:Convergent | Simulink:masks:Floor | Simulink:masks:Nearest | Simulink:masks:Round | Simulink:masks:Simplest | Simulink:masks:Zero
      mask Display: dpoly(NumCoefVec,[1 DenCoefVec],'z-')
  Transfer Fcn Direct Form II Time Varying : Subsystem  mask(Transfer Fcn Direct Form II Time Varying){vinit=0.0, RndMeth=Floor, DoSatur=off}
      mask prompts: vinit "Simulink:masks:InitialCondition_MP"; RndMeth "Simulink:masks:IntegerRoundingMode_MP"; DoSatur "Simulink:masks:SaturateToMaxOrMinWhenOverflowsOccur_MP"
      mask help: Simulink:masks:TransferFcnDirectFormIITimeVarying_MD
      mask init:
      | blkH = gcbh;
      | blkName = getfullname(blkH);
      | 
      | vRndMeth = get_param(blkH,'RndMeth');
      | vDoSatur = get_param(blkH,'DoSatur');
      | set_param([blkName,'/Dot1'],'RndMeth',vRndMeth, ...
      | 	'DoSatur',vDoSatur);
      | set_param([blkName,'/Dot2'],'RndMeth',vRndMeth, ...
      | 	'DoSatur',vDoSatur);
      | set_param([blkName,'/Downcast'],'RndMeth',vRndMeth, ...
      | 	'DoSatur',vDoSatur);
      | set_param([blkName,'/Downcast1'],'RndMeth',vRndMeth, ...
      | 	'DoSatur',vDoSatur);
      | set_param([blkName,'/Sum'],'RndMeth',vRndMeth, ...
      | 	'DoSatur',vDoSatur);
      mask TypeOptions RndMeth: Simulink:masks:Ceiling | Simulink:masks:Convergent | Simulink:masks:Floor | Simulink:masks:Nearest | Simulink:masks:Round | Simulink:masks:Simplest | Simulink:masks:Zero
      mask Display: fprintf('Direct\nForm II')
  Unit Delay Enabled : Subsystem  mask(Unit Delay Enabled){vinit=0.0, tsamp=-1}
      mask prompts: vinit "Simulink:masks:InitialCondition_MP"; tsamp "Simulink:masks:SampleTime_MP"
      mask help: Simulink:masks:UnitDelayEnabled_MD
      mask Display: dpoly(1,[1 0],'z')
  Unit Delay Enabled External IC : Subsystem  mask(Unit Delay Enabled External Initial Condition){tsamp=-1}
      mask prompts: tsamp "Simulink:masks:SampleTime_MP"
      mask help: Simulink:masks:UnitDelayEnabledExternalInitialCondition_MD
      mask Display: dpoly(1,[1 0],'z')
  Unit Delay Enabled Resettable : Subsystem  mask(Unit Delay Enabled Resettable){vinit=0.0, tsamp=-1}
      mask prompts: vinit "Simulink:masks:InitialCondition_MP"; tsamp "Simulink:masks:SampleTime_MP"
      mask help: Simulink:masks:UnitDelayEnabledResettable_MD
      mask Display: dpoly(1,[1 0],'z')
  Unit Delay Enabled Resettable External IC : Subsystem  mask(Unit Delay Enabled Resettable External Initial Condition){tsamp=-1}
      mask prompts: tsamp "Simulink:masks:SampleTime_MP"
      mask help: Simulink:masks:UnitDelayEnabledResettableExternalInitialCondition_MD
      mask Display: dpoly(1,[1 0],'z')
  Unit Delay External IC : Subsystem  mask(Unit Delay External Initial Condition){tsamp=-1}
      mask prompts: tsamp "Simulink:masks:SampleTime_MP"
      mask help: Simulink:masks:UnitDelayExternalInitialCondition_MD
      mask Display: dpoly(1,[1 0],'z')
  Unit Delay Resettable : Subsystem  mask(Unit Delay Resettable){vinit=0.0, tsamp=-1}
      mask prompts: vinit "Simulink:masks:InitialCondition_MP"; tsamp "Simulink:masks:SampleTime_MP"
      mask help: Simulink:masks:UnitDelayResettable_MD
      mask Display: dpoly(1,[1 0],'z')
  Unit Delay Resettable External IC : Subsystem  mask(Unit Delay Resettable External Initial Condition){tsamp=-1}
      mask prompts: tsamp "Simulink:masks:SampleTime_MP"
      mask help: Simulink:masks:UnitDelayResettableExternalInitialCondition_MD
      mask Display: dpoly(1,[1 0],'z')
  Unit Delay With Preview Enabled : Subsystem  mask(Unit Delay With Preview Enabled){vinit=0.0, tsamp=-1}
      mask prompts: vinit "Simulink:masks:InitialCondition_MP"; tsamp "Simulink:masks:SampleTime_MP"
      mask help: Simulink:masks:UnitDelayWithPreviewEnabled_MD
      mask Display:
      | plot([NaN 0.1 0.13 0.1 NaN 0.1 0.13 0.1 NaN 0.1 0.13 0.1 NaN -0.05 0.025 0.075 0.13 NaN -0.05 0.025 0.075 0.13 NaN 0.13 0.13 0.4475 0.4475 0.13 NaN 0.4475 0.4975 0.5525 0.5225 0.5525 0.5225 NaN 0.4475 0.4975 1.05 NaN 0.5525 0.5525 0.87 0.87 0.5525 NaN 0.71125 0.71125 NaN 0.6525 0.77 NaN 0.6525 0.77 0.6525 0.77 NaN 0.87 0.92 1.05 NaN 0.92 0.92 0.075 0.075 0.13],[NaN 0.846666666666667 0.816666666666667 0.786666666666667 NaN 0.58 0.55 0.52 NaN 0.313333333333333 0.283333333333333 0.253333333333333 NaN 0.75 0.75 0.816666666666667 0.816666666666667 NaN 0.25 0.25 0.55 0.55 NaN 0.15 0.95 0.95 0.15 0.15 NaN 0.55 0.35 0.35 0.38 0.35 0.32 NaN 0.55 0.75 0.75 NaN 0.15 0.55 0.55 0.15 0.15 NaN 0.5 0.4 NaN 0.35 0.35 NaN 0.3 0.3 0.2 0.2 NaN 0.35 0.25 0.25 NaN 0.25 0.05 0.05 0.283333333333333 0.283333333333333]);
      | text(0.23,0.806666666666667,'u');
      | text(0.23,0.54,'E');
  Unit Delay With Preview Enabled Resettable : Subsystem  mask(Unit Delay With Preview Enabled Resettable){vinit=0.0, tsamp=-1}
      mask prompts: vinit "Simulink:masks:InitialCondition_MP"; tsamp "Simulink:masks:SampleTime_MP"
      mask help: Simulink:masks:UnitDelayWithPreviewEnabledResettable_MD
      mask Display:
      | plot([NaN 0.1 0.13 0.1 NaN 0.1 0.13 0.1 NaN 0.1 0.13 0.1 NaN 0.1 0.13 0.1 NaN -0.05 0.025 0.075 0.13 NaN -0.05 0.025 0.075 0.13 NaN -0.05 0.025 0.075 0.13 NaN 0.13 0.13 0.4475 0.4475 0.13 NaN 0.4475 0.4975 0.5525 0.5225 0.5525 0.5225 NaN 0.4475 0.4975 1.05 NaN 0.5525 0.5525 0.87 0.87 0.5525 NaN 0.71125 0.71125 NaN 0.6525 0.77 NaN 0.6525 0.77 0.6525 0.77 NaN 0.87 0.92 1.05 NaN 0.92 0.92 0.075 0.075 0.13],[NaN 0.88 0.85 0.82 NaN 0.68 0.65 0.62 NaN 0.48 0.45 0.42 NaN 0.28 0.25 0.22 NaN 0.833333333333333 0.833333333333333 0.85 0.85 NaN 0.5 0.5 0.65 0.65 NaN 0.166666666666667 0.166666666666667 0.45 0.45 NaN 0.15 0.95 0.95 0.15 0.15 NaN 0.55 0.35 0.35 0.38 0.35 0.32 NaN 0.55 0.75 0.75 NaN 0.15 0.55 0.55 0.15 0.15 NaN 0.5 0.4 NaN 0.35 0.35 NaN 0.3 0.3 0.2 0.2 NaN 0.35 0.25 0.25 NaN 0.25 0.05 0.05 0.25 0.25]);
      | text(0.23,0.84,'u');
      | text(0.23,0.64,'E');
      | text(0.23,0.44,'R');
  Unit Delay With Preview Enabled Resettable External RV : Subsystem  mask(Unit Delay With Preview Enabled Resettable External RV){vinit=0.0, tsamp=-1}
      mask prompts: vinit "Simulink:masks:InitialCondition_MP"; tsamp "Simulink:masks:SampleTime_MP"
      mask help: Simulink:masks:UnitDelayWithPreviewEnabledResettableExternalRV_MD
      mask Display:
      | plot([NaN 0.1 0.13 0.1 NaN 0.1 0.13 0.1 NaN 0.1 0.13 0.1 NaN 0.1 0.13 0.1 NaN 0.1 0.13 0.1 NaN -0.05 0.025 0.075 0.13 NaN -0.05 0.025 0.075 0.13 NaN -0.05 0.025 0.075 0.13 NaN -0.05 0.025 0.075 0.13 NaN 0.13 0.13 0.4475 0.4475 0.13 NaN 0.4475 0.4975 0.5525 0.5225 0.5525 0.5225 NaN 0.4475 0.4975 1.05 NaN 0.5525 0.5525 0.87 0.87 0.5525 NaN 0.71125 0.71125 NaN 0.6525 0.77 NaN 0.6525 0.77 0.6525 0.77 NaN 0.87 0.92 1.05 NaN 0.92 0.92 0.075 0.075 0.13],[NaN 0.9 0.87 0.84 NaN 0.74 0.71 0.68 NaN 0.58 0.55 0.52 NaN 0.42 0.39 0.36 NaN 0.26 0.23 0.2 NaN 0.875 0.875 0.87 0.87 NaN 0.625 0.625 0.71 0.71 NaN 0.375 0.375 0.55 0.55 NaN 0.125 0.125 0.39 0.39 NaN 0.15 0.95 0.95 0.15 0.15 NaN 0.55 0.35 0.35 0.38 0.35 0.32 NaN 0.55 0.75 0.75 NaN 0.15 0.55 0.55 0.15 0.15 NaN 0.5 0.4 NaN 0.35 0.35 NaN 0.3 0.3 0.2 0.2 NaN 0.35 0.25 0.25 NaN 0.25 0.05 0.05 0.23 0.23]);
      | text(0.23,0.86,'u');
      | text(0.23,0.7,'E');
      | text(0.23,0.54,'R');
      | text(0.23,0.38,'RV');
  Unit Delay With Preview Resettable : Subsystem  mask(Unit Delay With Preview Resettable){vinit=0.0, tsamp=-1}
      mask prompts: vinit "Simulink:masks:InitialCondition_MP"; tsamp "Simulink:masks:SampleTime_MP"
      mask help: Simulink:masks:UnitDelayWithPreviewResettable_MD
      mask Display:
      | plot([NaN 0.1 0.13 0.1 NaN 0.1 0.13 0.1 NaN -0.05 0.025 0.075 0.13 NaN -0.05 0.025 0.075 0.13 NaN 0.13 0.13 0.4475 0.4475 0.13 NaN 0.4475 0.4975 0.5525 0.5225 0.5525 0.5225 NaN 0.4475 0.4975 1.05 NaN 0.5525 0.5525 0.87 0.87 0.5525 NaN 0.71125 0.71125 NaN 0.6525 0.77 NaN 0.6525 0.77 0.6525 0.77 NaN 0.87 0.92 1.05],[NaN 0.755 0.725 0.695 NaN 0.305 0.275 0.245 NaN 0.75 0.75 0.725 0.725 NaN 0.25 0.25 0.275 0.275 NaN 0.0499999999999999 0.95 0.95 0.0499999999999999 0.0499999999999999 NaN 0.5 0.275 0.275 0.305 0.275 0.245 NaN 0.5 0.75 0.75 NaN 0.0499999999999999 0.5 0.5 0.0499999999999999 0.0499999999999999 NaN 0.45 0.325 NaN 0.275 0.275 NaN 0.225 0.225 0.0999999999999999 0.0999999999999999 NaN 0.275 0.25 0.25]);
      | text(0.23,0.715,'u');
      | text(0.23,0.265,'R');
  Unit Delay With Preview Resettable External RV : Subsystem  mask(Unit Delay With Preview Resettable External RV){vinit=0.0, tsamp=-1}
      mask prompts: vinit "Simulink:masks:InitialCondition_MP"; tsamp "Simulink:masks:SampleTime_MP"
      mask help: Simulink:masks:UnitDelayWithPreviewResettableExternalRV_MD
      mask Display:
      | plot([NaN 0.1 0.13 0.1 NaN 0.1 0.13 0.1 NaN 0.1 0.13 0.1 NaN -0.05 0.025 0.075 0.13 NaN -0.05 0.025 0.075 0.13 NaN -0.05 0.025 0.075 0.13 NaN 0.13 0.13 0.4475 0.4475 0.13 NaN 0.4475 0.4975 0.5525 0.5225 0.5525 0.5225 NaN 0.4475 0.4975 1.05 NaN 0.5525 0.5525 0.87 0.87 0.5525 NaN 0.71125 0.71125 NaN 0.6525 0.77 NaN 0.6525 0.77 0.6525 0.77 NaN 0.87 0.92 1.05],[NaN 0.83 0.8 0.77 NaN 0.53 0.5 0.47 NaN 0.23 0.2 0.17 NaN 0.833333333333333 0.833333333333333 0.8 0.8 NaN 0.5 0.5 0.5 0.5 NaN 0.166666666666667 0.166666666666667 0.2 0.2 NaN 0.0499999999999999 0.95 0.95 0.0499999999999999 0.0499999999999999 NaN 0.5 0.275 0.275 0.305 0.275 0.245 NaN 0.5 0.75 0.75 NaN 0.0499999999999999 0.5 0.5 0.0499999999999999 0.0499999999999999 NaN 0.45 0.325 NaN 0.275 0.275 NaN 0.225 0.225 0.0999999999999999 0.0999999999999999 NaN 0.275 0.25 0.25]);
      | text(0.23,0.79,'u');
      | text(0.23,0.49,'R');
      | text(0.23,0.19,'RV');

== system simulink/Additional Math & Discrete/Additional Math: Increment - Decrement ==
  note: Increment/Decrement
  Decrement Real World : Subsystem  mask(Real World Value Decrement){}
      mask help: Simulink:masks:RealWorldValueDecrement_MD
      mask Display: disp('V--')
  Decrement Stored Integer : Subsystem  mask(Stored Integer Value Decrement){}
      mask help: Simulink:masks:StoredIntegerValueDecrement_MD
      mask Display: disp('Q--')
  Decrement To Zero : Subsystem  mask(Decrement To Zero){}
      mask help: Simulink:masks:DecrementToZero_MD
      mask Display: fprintf('max( V--, 0 )');
  Decrement Time To Zero : Subsystem  mask(Decrement Time To Zero){}
      mask help: Simulink:masks:DecrementTimeToZero_MD
      mask Display: fprintf('max( V-Ts, 0 )');
  Increment Real World : Subsystem  mask(Real World Value Increment){}
      mask help: Simulink:masks:RealWorldValueIncrement_MD
      mask Display: disp('V++')
  Increment Stored Integer : Subsystem  mask(Stored Integer Value Increment){}
      mask help: Simulink:masks:StoredIntegerValueIncrement_MD
      mask Display: disp('Q++')

== system simulink/Commonly Used Blocks/Subsystem ==
  In1 : Inport
  Out1 : Outport
  wires:
  In1/1 -> Out1/1

== system simulink/Continuous/PID Controller ==
  u : Inport
  Derivative Gain : Gain  DisableCoverage=on  Gain=D  ParamMin=DParamMin  ParamMax=DParamMax  ParamDataTypeStr=DParamDataTypeStr  OutMin=DOutMin  OutMax=DOutMax  OutDataTypeStr=DOutDataTypeStr
  Filter : Integrator  DisableCoverage=on  InitialCondition=InitialConditionForFilter
  Filter Coefficient : Gain  Gain=N  ParamMin=NParamMin  ParamMax=NParamMax  ParamDataTypeStr=NParamDataTypeStr  OutMin=NOutMin  OutMax=NOutMax  OutDataTypeStr=NOutDataTypeStr
  Integral Gain : Gain  DisableCoverage=on  Gain=I  ParamMin=IParamMin  ParamMax=IParamMax  ParamDataTypeStr=IParamDataTypeStr  OutMin=IOutMin  OutMax=IOutMax  OutDataTypeStr=IOutDataTypeStr
  Integrator : Integrator  InitialCondition=InitialConditionForIntegrator
  Proportional Gain : Gain  Gain=P  ParamMin=PParamMin  ParamMax=PParamMax  ParamDataTypeStr=PParamDataTypeStr  OutMin=POutMin  OutMax=POutMax  OutDataTypeStr=POutDataTypeStr
  Sum : Sum  Inputs=+++  AccumDataTypeStr=SumAccumDataTypeStr  OutMin=SumOutMin  OutMax=SumOutMax  OutDataTypeStr=SumOutDataTypeStr
  SumD : Sum  DisableCoverage=on  Inputs=|+-  AccumDataTypeStr=SumDAccumDataTypeStr  OutMin=SumDOutMin  OutMax=SumDOutMax  OutDataTypeStr=SumDOutDataTypeStr
  y : Outport  InitialOutput=0
  wires:
  u/1 -> Proportional Gain/1, Integral Gain/1, Derivative Gain/1
  Proportional Gain/1 -> Sum/1
  Integral Gain/1 -> Integrator/1
  Derivative Gain/1 -> SumD/1
  SumD/1 -> Filter Coefficient/1
  Filter Coefficient/1 -> Filter/1, Sum/3
  Filter/1 -> SumD/2
  Integrator/1 -> Sum/2
  Sum/1 -> y/1
